simulink model "Closed_Loop_TF_Sin"  (R2023a)
settings: Solver=VariableStepAuto  StartTime=0.0  StopTime=10.0  RelTol=1e-6
undefined symbols (not defined in the file): a, b, d, K, M, w
settings Model: Creator=m260477  LastModifiedBy=m260477

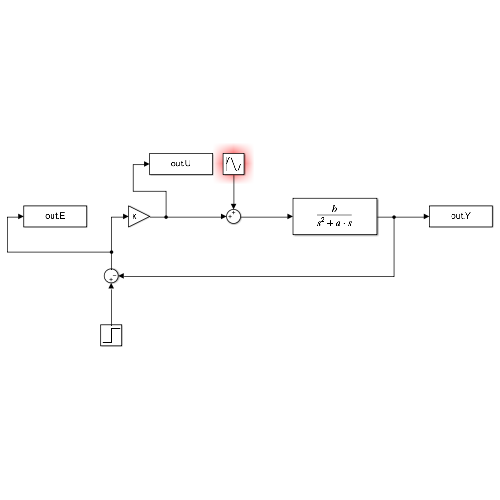
[thumbnail: Simulink's stored preview of the top-level diagram]
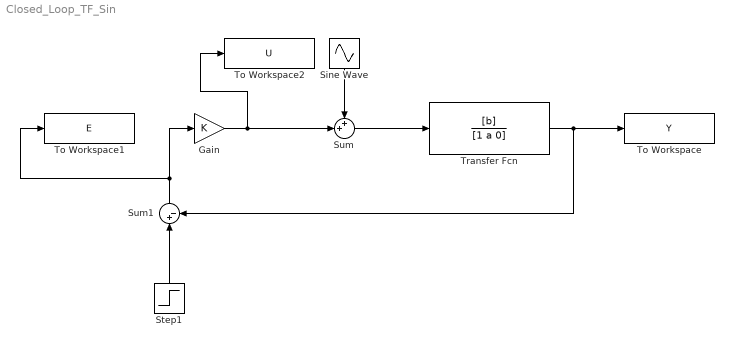
== system Closed_Loop_TF_Sin ==
  Gain : Gain  Gain=K
  Sine Wave : Sin  Amplitude=d  Frequency=w  SampleTime=0
  Step1 : Step  Time=0  After=M  SampleTime=0
  Sum : Sum  Inputs=++|
  Sum1 : Sum  Inputs=|+-
  To Workspace : ToWorkspace  VariableName=Y  SaveFormat=Timeseries  SampleTime=-1
  To Workspace1 : ToWorkspace  VariableName=E  SaveFormat=Timeseries  SampleTime=-1
  To Workspace2 : ToWorkspace  VariableName=U  SaveFormat=Timeseries  SampleTime=-1
  Transfer Fcn : TransferFcn  Numerator=[b]  Denominator=[1 a 0]
  wires:
  Step1/1 -> Sum1/1
  Sum/1 -> Transfer Fcn/1
  Sine Wave/1 -> Sum/1
  Sum1/1 -> To Workspace1/1, Gain/1
  Gain/1 -> To Workspace2/1, Sum/2
  Transfer Fcn/1 -> To Workspace/1, Sum1/2
